simulink subsystem "station1"  (R2024b)
settings: Solver=VariableStepAuto  StartTime=0.0  StopTime=10.0  RelTol=1e-3
undefined symbols (not defined in the file): DiscIntNeverNeededParam, DPL1ph, h, Half, R3, ResistanceM, Rt4, simetran, Ts, Zm
libraries: ee_lib x102, fl_lib x54, nesl_utility x45, simulink x7
(part 3 of 3)

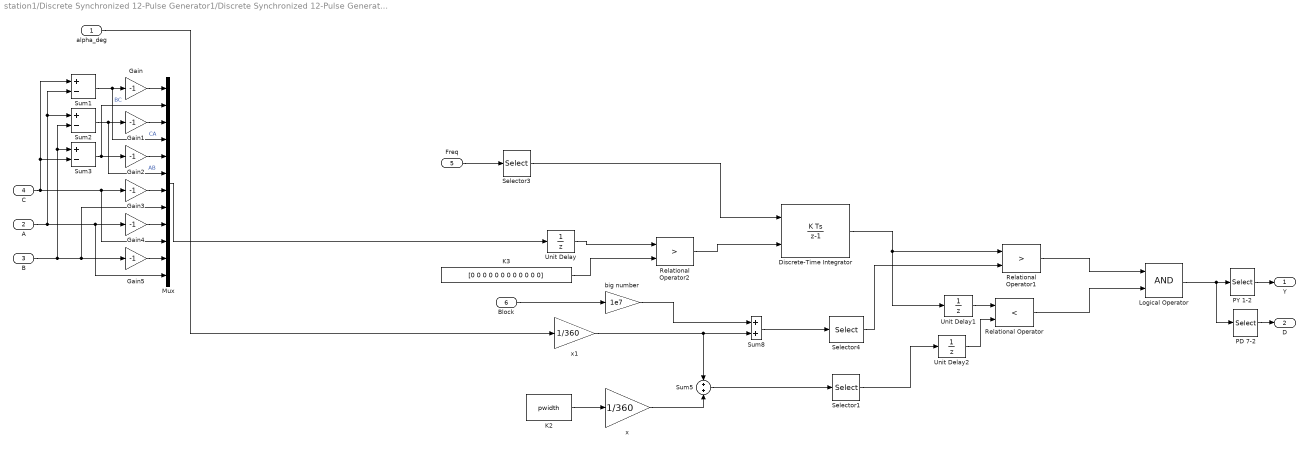
== system station1/Discrete Synchronized 12-Pulse Generator1/Discrete Synchronized 12-Pulse Generator2 ==
  alpha_deg : Inport
  A : Inport  Port=2
  B : Inport  Port=3
  C : Inport  Port=4
  Freq : Inport  Port=5
  Block : Inport  Port=6
  Discrete-Time Integrator : DiscreteIntegrator  ExternalReset=rising  SampleTime=Ts  ICPrevOutput=DiscIntNeverNeededParam  ICPrevScaledInput=DiscIntNeverNeededParam
  Gain{,1..5} (6 alike) : Gain  Gain=-1  SaturateOnIntegerOverflow=on  OutDataTypeStr=Inherit: Same as input  ParamDataTypeStr=Inherit: Same as input
  K2 : Constant  Value=pwidth
  K3 : Constant  Value=[0 0 0 0 0 0 0 0 0 0 0 0]
  Logical Operator : Logic  AllPortsSameDT=off  OutDataTypeStr=boolean
  Mux : Mux  Inputs=12
  PD 7-2 : Selector  InputPortWidth=12  IndexOptions=Index vector (dialog)  Indices=7:12  OutputSizes=1
  PY 1-2 : Selector  InputPortWidth=12  IndexOptions=Index vector (dialog)  Indices=1:6  OutputSizes=1
  Relational Operator : RelationalOperator  Operator=<  OutDataTypeStr=boolean  RndMeth=Simplest  InputSameDT=off
  Relational Operator1 : RelationalOperator  Operator=>  OutDataTypeStr=boolean  RndMeth=Simplest  InputSameDT=off
  Relational Operator2 : RelationalOperator  Operator=>  OutDataTypeStr=boolean  RndMeth=Simplest  InputSameDT=off
  Selector1 : Selector  InputPortWidth=1  IndexOptions=Index vector (dialog)  Indices=[1 1 1 1 1 1 1 1 1 1 1 1]  OutputSizes=1
  Selector3 : Selector  InputPortWidth=1  IndexOptions=Index vector (dialog)  Indices=[1 1 1 1 1 1 1 1 1 1 1 1]  OutputSizes=1
  Selector4 : Selector  InputPortWidth=1  IndexOptions=Index vector (dialog)  Indices=[1 1 1 1 1 1 1 1 1 1 1 1]  OutputSizes=1
  Sum1 : Sum  Inputs=+-  InputSameDT=on  SaturateOnIntegerOverflow=on  OutDataTypeStr=Inherit: Same as first input
  Sum2 : Sum  Inputs=+-  InputSameDT=on  SaturateOnIntegerOverflow=on  OutDataTypeStr=Inherit: Same as first input
  Sum3 : Sum  Inputs=+-  InputSameDT=on  SaturateOnIntegerOverflow=on  OutDataTypeStr=Inherit: Same as first input
  Sum5 : Sum  InputSameDT=on  SaturateOnIntegerOverflow=on  OutDataTypeStr=Inherit: Same as first input
  Sum8 : Sum  InputSameDT=on  SaturateOnIntegerOverflow=on  OutDataTypeStr=Inherit: Same as first input
  Unit Delay : UnitDelay  InitialCondition=-1  SampleTime=Ts  HasFrameUpgradeWarning=on
  Unit Delay1 : UnitDelay  InitialCondition=-1  SampleTime=Ts  HasFrameUpgradeWarning=on
  Unit Delay2 : UnitDelay  InitialCondition=-1  SampleTime=Ts  HasFrameUpgradeWarning=on
  big number : Gain  Gain=1e7  SaturateOnIntegerOverflow=on  OutDataTypeStr=Inherit: Same as input  ParamDataTypeStr=Inherit: Same as input
  x : Gain  Gain=1/360  SaturateOnIntegerOverflow=on  OutDataTypeStr=Inherit: Same as input  ParamDataTypeStr=Inherit: Same as input
  x1 : Gain  Gain=1/360  SaturateOnIntegerOverflow=on  OutDataTypeStr=Inherit: Same as input  ParamDataTypeStr=Inherit: Same as input
  Y : Outport  InitialOutput=0
  D : Outport  Port=2  InitialOutput=0
  wires:
  Unit Delay2/1 -> Relational Operator/2
  Unit Delay1/1 -> Relational Operator/1
  Freq/1 -> Selector3/1
  Gain2/1 -> Mux/5
  Gain1/1 -> Mux/3
  Gain/1 -> Mux/1
  Sum1/1 -> Gain/1, Mux/4  "CA"
  Sum2/1 -> Gain1/1, Mux/6  "AB"
  Sum3/1 -> Gain2/1, Mux/2  "BC"
  Gain3/1 -> Mux/7
  Gain4/1 -> Mux/9
  Gain5/1 -> Mux/11
  C/1 -> Gain3/1, Mux/10, Sum1/1, Sum3/2
  A/1 -> Gain4/1, Mux/12, Sum2/1, Sum1/2
  B/1 -> Gain5/1, Mux/8, Sum3/1, Sum2/2
  Block/1 -> big number/1
  Selector3/1 -> Discrete-Time Integrator/1
  big number/1 -> Sum8/1
  Selector1/1 -> Unit Delay2/1
  Logical Operator/1 -> PD 7-2/1, PY 1-2/1
  Sum5/1 -> Selector1/1
  Discrete-Time Integrator/1 -> Relational Operator1/1, Unit Delay1/1
  Mux/1 -> Unit Delay/1
  K3/1 -> Relational Operator2/2
  Relational Operator1/1 -> Logical Operator/1
  Relational Operator/1 -> Logical Operator/2
  x/1 -> Sum5/2
  K2/1 -> x/1
  Relational Operator2/1 -> Discrete-Time Integrator/2
  alpha_deg/1 -> x1/1
  Unit Delay/1 -> Relational Operator2/1
  Sum8/1 -> Selector4/1
  PD 7-2/1 -> D/1
  PY 1-2/1 -> Y/1
  x1/1 -> Sum8/2, Sum5/1
  Selector4/1 -> Relational Operator1/2

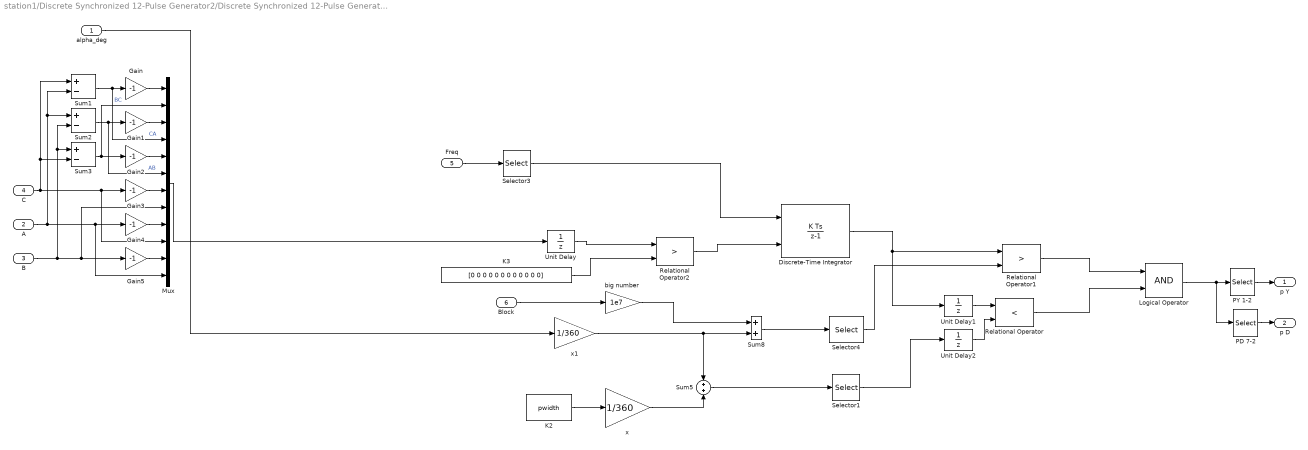
== system station1/Discrete Synchronized 12-Pulse Generator2/Discrete Synchronized 12-Pulse Generator2 ==
  alpha_deg : Inport
  A : Inport  Port=2
  B : Inport  Port=3
  C : Inport  Port=4
  Freq : Inport  Port=5
  Block : Inport  Port=6
  Discrete-Time Integrator : DiscreteIntegrator  ExternalReset=rising  SampleTime=Ts  ICPrevOutput=DiscIntNeverNeededParam  ICPrevScaledInput=DiscIntNeverNeededParam
  Gain{,1..5} (6 alike) : Gain  Gain=-1  SaturateOnIntegerOverflow=on  OutDataTypeStr=Inherit: Same as input  ParamDataTypeStr=Inherit: Same as input
  K2 : Constant  Value=pwidth
  K3 : Constant  Value=[0 0 0 0 0 0 0 0 0 0 0 0]
  Logical Operator : Logic  AllPortsSameDT=off  OutDataTypeStr=boolean
  Mux : Mux  Inputs=12
  PD 7-2 : Selector  InputPortWidth=12  IndexOptions=Index vector (dialog)  Indices=7:12  OutputSizes=1
  PY 1-2 : Selector  InputPortWidth=12  IndexOptions=Index vector (dialog)  Indices=1:6  OutputSizes=1
  Relational Operator : RelationalOperator  Operator=<  OutDataTypeStr=boolean  RndMeth=Simplest  InputSameDT=off
  Relational Operator1 : RelationalOperator  Operator=>  OutDataTypeStr=boolean  RndMeth=Simplest  InputSameDT=off
  Relational Operator2 : RelationalOperator  Operator=>  OutDataTypeStr=boolean  RndMeth=Simplest  InputSameDT=off
  Selector1 : Selector  InputPortWidth=1  IndexOptions=Index vector (dialog)  Indices=[1 1 1 1 1 1 1 1 1 1 1 1]  OutputSizes=1
  Selector3 : Selector  InputPortWidth=1  IndexOptions=Index vector (dialog)  Indices=[1 1 1 1 1 1 1 1 1 1 1 1]  OutputSizes=1
  Selector4 : Selector  InputPortWidth=1  IndexOptions=Index vector (dialog)  Indices=[1 1 1 1 1 1 1 1 1 1 1 1]  OutputSizes=1
  Sum1 : Sum  Inputs=+-  InputSameDT=on  SaturateOnIntegerOverflow=on  OutDataTypeStr=Inherit: Same as first input
  Sum2 : Sum  Inputs=+-  InputSameDT=on  SaturateOnIntegerOverflow=on  OutDataTypeStr=Inherit: Same as first input
  Sum3 : Sum  Inputs=+-  InputSameDT=on  SaturateOnIntegerOverflow=on  OutDataTypeStr=Inherit: Same as first input
  Sum5 : Sum  InputSameDT=on  SaturateOnIntegerOverflow=on  OutDataTypeStr=Inherit: Same as first input
  Sum8 : Sum  InputSameDT=on  SaturateOnIntegerOverflow=on  OutDataTypeStr=Inherit: Same as first input
  Unit Delay : UnitDelay  InitialCondition=-1  SampleTime=Ts  HasFrameUpgradeWarning=on
  Unit Delay1 : UnitDelay  InitialCondition=-1  SampleTime=Ts  HasFrameUpgradeWarning=on
  Unit Delay2 : UnitDelay  InitialCondition=-1  SampleTime=Ts  HasFrameUpgradeWarning=on
  big number : Gain  Gain=1e7  SaturateOnIntegerOverflow=on  OutDataTypeStr=Inherit: Same as input  ParamDataTypeStr=Inherit: Same as input
  x : Gain  Gain=1/360  SaturateOnIntegerOverflow=on  OutDataTypeStr=Inherit: Same as input  ParamDataTypeStr=Inherit: Same as input
  x1 : Gain  Gain=1/360  SaturateOnIntegerOverflow=on  OutDataTypeStr=Inherit: Same as input  ParamDataTypeStr=Inherit: Same as input
  p Y : Outport  InitialOutput=0
  p D : Outport  Port=2  InitialOutput=0
  wires:
  Selector4/1 -> Relational Operator1/2
  x1/1 -> Sum5/1, Sum8/2
  PY 1-2/1 -> p Y/1
  PD 7-2/1 -> p D/1
  Sum8/1 -> Selector4/1
  Unit Delay/1 -> Relational Operator2/1
  alpha_deg/1 -> x1/1
  Relational Operator2/1 -> Discrete-Time Integrator/2
  K2/1 -> x/1
  x/1 -> Sum5/2
  Relational Operator/1 -> Logical Operator/2
  Relational Operator1/1 -> Logical Operator/1
  K3/1 -> Relational Operator2/2
  Mux/1 -> Unit Delay/1
  Discrete-Time Integrator/1 -> Unit Delay1/1, Relational Operator1/1
  Sum5/1 -> Selector1/1
  Logical Operator/1 -> PY 1-2/1, PD 7-2/1
  Selector1/1 -> Unit Delay2/1
  big number/1 -> Sum8/1
  Selector3/1 -> Discrete-Time Integrator/1
  Block/1 -> big number/1
  B/1 -> Sum2/2, Sum3/1, Mux/8, Gain5/1
  A/1 -> Sum1/2, Sum2/1, Mux/12, Gain4/1
  C/1 -> Sum3/2, Sum1/1, Mux/10, Gain3/1
  Gain5/1 -> Mux/11
  Gain4/1 -> Mux/9
  Gain3/1 -> Mux/7
  Sum3/1 -> Mux/2, Gain2/1  "BC"
  Sum2/1 -> Mux/6, Gain1/1  "AB"
  Sum1/1 -> Mux/4, Gain/1  "CA"
  Gain/1 -> Mux/1
  Gain1/1 -> Mux/3
  Gain2/1 -> Mux/5
  Freq/1 -> Selector3/1
  Unit Delay1/1 -> Relational Operator/1
  Unit Delay2/1 -> Relational Operator/2

== system station1/Filters 60Hz8/High-pass filter ==
  CC : fl_lib/Electrical/Electrical Elements/Capacitor  c=C1 F  r=0 Ohm  g=0 1/Ohm  i_specify=off  i_priority=None  i=0 A  i_nominal_specify=off  i_nominal_value=1  i_nominal_unit=A  v_specify=off  v_priority=None  v=0 V  v_nominal_specify=off  v_nominal_value=1  v_nominal_unit=V  vc_specify=off  vc_priority=High  vc=0 V  vc_nominal_specify=off  vc_nominal_value=1  vc_nominal_unit=V
  CC1 : fl_lib/Electrical/Electrical Elements/Capacitor  c=C1 F  r=0 Ohm  g=0 1/Ohm  i_specify=off  i_priority=None  i=0 A  i_nominal_specify=off  i_nominal_value=1  i_nominal_unit=A  v_specify=off  v_priority=None  v=0 V  v_nominal_specify=off  v_nominal_value=1  v_nominal_unit=V  vc_specify=off  vc_priority=High  vc=0 V  vc_nominal_specify=off  vc_nominal_value=1  vc_nominal_unit=V
  CC2 : fl_lib/Electrical/Electrical Elements/Capacitor  c=C1 F  r=0 Ohm  g=0 1/Ohm  i_specify=off  i_priority=None  i=0 A  i_nominal_specify=off  i_nominal_value=1  i_nominal_unit=A  v_specify=off  v_priority=None  v=0 V  v_nominal_specify=off  v_nominal_value=1  v_nominal_unit=V  vc_specify=off  vc_priority=High  vc=0 V  vc_nominal_specify=off  vc_nominal_value=1  vc_nominal_unit=V
  Electrical Reference : fl_lib/Electrical/Electrical Elements/Electrical Reference
  Electrical Reference1 : fl_lib/Electrical/Electrical Elements/Electrical Reference
  Electrical Reference2 : fl_lib/Electrical/Electrical Elements/Electrical Reference
  Phase Splitter : ee_lib/Connectors & References/Phase Splitter
  RL parallel : fl_lib/Electrical/Electrical Elements/Inductor  l=L2 H  r=0 Ohm  g=1/R3 1/Ohm  i_specify=off  i_priority=None  i=0 A  i_nominal_specify=off  i_nominal_value=1  i_nominal_unit=A  v_specify=off  v_priority=None  v=0 V  v_nominal_specify=off  v_nominal_value=1  v_nominal_unit=V  i_L_specify=off  i_L_priority=High  i_L=0 A  i_L_nominal_specify=off  i_L_nominal_value=1  i_L_nominal_unit=A
  RL parallel1 : fl_lib/Electrical/Electrical Elements/Inductor  l=L2 H  r=0 Ohm  g=1/R3 1/Ohm  i_specify=off  i_priority=None  i=0 A  i_nominal_specify=off  i_nominal_value=1  i_nominal_unit=A  v_specify=off  v_priority=None  v=0 V  v_nominal_specify=off  v_nominal_value=1  v_nominal_unit=V  i_L_specify=off  i_L_priority=High  i_L=0 A  i_L_nominal_specify=off  i_L_nominal_value=1  i_L_nominal_unit=A
  RL parallel2 : fl_lib/Electrical/Electrical Elements/Inductor  l=L2 H  r=0 Ohm  g=1/R3 1/Ohm  i_specify=off  i_priority=None  i=0 A  i_nominal_specify=off  i_nominal_value=1  i_nominal_unit=A  v_specify=off  v_priority=None  v=0 V  v_nominal_specify=off  v_nominal_value=1  v_nominal_unit=V  i_L_specify=off  i_L_priority=High  i_L=0 A  i_L_nominal_specify=off  i_L_nominal_value=1  i_L_nominal_unit=A
  abc : PMIOPort  Side=Right
  connections:
  CC2/LConn1 -- Phase Splitter/RConn3
  CC/LConn1 -- Phase Splitter/RConn1
  Phase Splitter/RConn2 -- CC1/LConn1
  Phase Splitter/LConn1 -- abc/RConn1
  RL parallel/LConn1 -- CC/RConn1
  RL parallel/RConn1 -- Electrical Reference/LConn1
  CC1/RConn1 -- RL parallel1/LConn1
  RL parallel1/RConn1 -- Electrical Reference1/LConn1
  RL parallel2/RConn1 -- Electrical Reference2/LConn1
  CC2/RConn1 -- RL parallel2/LConn1

== system station1/Filters 60Hz8/tuned filter 11th ==
  Electrical Reference : fl_lib/Electrical/Electrical Elements/Electrical Reference
  Electrical Reference1 : fl_lib/Electrical/Electrical Elements/Electrical Reference
  Electrical Reference2 : fl_lib/Electrical/Electrical Elements/Electrical Reference
  Inductor : fl_lib/Electrical/Electrical Elements/Inductor  l=L1 H  r=R2 Ohm  g=1e-9 1/Ohm  i_specify=off  i_priority=None  i=0 A  i_nominal_specify=off  i_nominal_value=1  i_nominal_unit=A  v_specify=off  v_priority=None  v=0 V  v_nominal_specify=off  v_nominal_value=1  v_nominal_unit=V  i_L_specify=off  i_L_priority=High  i_L=0 A  i_L_nominal_specify=off  i_L_nominal_value=1  i_L_nominal_unit=A
  Inductor1 : fl_lib/Electrical/Electrical Elements/Inductor  l=L1 H  r=R2 Ohm  g=1e-9 1/Ohm  i_specify=off  i_priority=None  i=0 A  i_nominal_specify=off  i_nominal_value=1  i_nominal_unit=A  v_specify=off  v_priority=None  v=0 V  v_nominal_specify=off  v_nominal_value=1  v_nominal_unit=V  i_L_specify=off  i_L_priority=High  i_L=0 A  i_L_nominal_specify=off  i_L_nominal_value=1  i_L_nominal_unit=A
  Inductor2 : fl_lib/Electrical/Electrical Elements/Inductor  l=L1 H  r=R2 Ohm  g=1e-9 1/Ohm  i_specify=off  i_priority=None  i=0 A  i_nominal_specify=off  i_nominal_value=1  i_nominal_unit=A  v_specify=off  v_priority=None  v=0 V  v_nominal_specify=off  v_nominal_value=1  v_nominal_unit=V  i_L_specify=off  i_L_priority=High  i_L=0 A  i_L_nominal_specify=off  i_L_nominal_value=1  i_L_nominal_unit=A
  Phase Splitter : ee_lib/Connectors & References/Phase Splitter
  RC : fl_lib/Electrical/Electrical Elements/Capacitor  c=C1 F  r=0 Ohm  g=0 1/Ohm  i_specify=off  i_priority=None  i=0 A  i_nominal_specify=off  i_nominal_value=1  i_nominal_unit=A  v_specify=off  v_priority=None  v=0 V  v_nominal_specify=off  v_nominal_value=1  v_nominal_unit=V  vc_specify=off  vc_priority=High  vc=0 V  vc_nominal_specify=off  vc_nominal_value=1  vc_nominal_unit=V
  RC1 : fl_lib/Electrical/Electrical Elements/Capacitor  c=C1 F  r=0 Ohm  g=0 1/Ohm  i_specify=off  i_priority=None  i=0 A  i_nominal_specify=off  i_nominal_value=1  i_nominal_unit=A  v_specify=off  v_priority=None  v=0 V  v_nominal_specify=off  v_nominal_value=1  v_nominal_unit=V  vc_specify=off  vc_priority=High  vc=0 V  vc_nominal_specify=off  vc_nominal_value=1  vc_nominal_unit=V
  RC2 : fl_lib/Electrical/Electrical Elements/Capacitor  c=C1 F  r=0 Ohm  g=0 1/Ohm  i_specify=off  i_priority=None  i=0 A  i_nominal_specify=off  i_nominal_value=1  i_nominal_unit=A  v_specify=off  v_priority=None  v=0 V  v_nominal_specify=off  v_nominal_value=1  v_nominal_unit=V  vc_specify=off  vc_priority=High  vc=0 V  vc_nominal_specify=off  vc_nominal_value=1  vc_nominal_unit=V
  abc : PMIOPort  Side=Right
  connections:
  Phase Splitter/LConn1 -- abc/RConn1
  RC2/LConn1 -- Phase Splitter/RConn3
  RC/LConn1 -- Phase Splitter/RConn1
  Phase Splitter/RConn2 -- RC1/LConn1
  RC2/RConn1 -- Inductor2/LConn1
  Inductor2/RConn1 -- Electrical Reference2/LConn1
  Inductor1/RConn1 -- Electrical Reference1/LConn1
  RC1/RConn1 -- Inductor1/LConn1
  Inductor/RConn1 -- Electrical Reference/LConn1
  Inductor/LConn1 -- RC/RConn1

== system station1/Filters 60Hz8/tuned filter 13th ==
  Electrical Reference : fl_lib/Electrical/Electrical Elements/Electrical Reference
  Electrical Reference1 : fl_lib/Electrical/Electrical Elements/Electrical Reference
  Electrical Reference2 : fl_lib/Electrical/Electrical Elements/Electrical Reference
  Inductor : fl_lib/Electrical/Electrical Elements/Inductor  l=L1 H  r=R2 Ohm  g=1e-9 1/Ohm  i_specify=off  i_priority=None  i=0 A  i_nominal_specify=off  i_nominal_value=1  i_nominal_unit=A  v_specify=off  v_priority=None  v=0 V  v_nominal_specify=off  v_nominal_value=1  v_nominal_unit=V  i_L_specify=off  i_L_priority=High  i_L=0 A  i_L_nominal_specify=off  i_L_nominal_value=1  i_L_nominal_unit=A
  Inductor1 : fl_lib/Electrical/Electrical Elements/Inductor  l=L1 H  r=R2 Ohm  g=1e-9 1/Ohm  i_specify=off  i_priority=None  i=0 A  i_nominal_specify=off  i_nominal_value=1  i_nominal_unit=A  v_specify=off  v_priority=None  v=0 V  v_nominal_specify=off  v_nominal_value=1  v_nominal_unit=V  i_L_specify=off  i_L_priority=High  i_L=0 A  i_L_nominal_specify=off  i_L_nominal_value=1  i_L_nominal_unit=A
  Inductor2 : fl_lib/Electrical/Electrical Elements/Inductor  l=L1 H  r=R2 Ohm  g=1e-9 1/Ohm  i_specify=off  i_priority=None  i=0 A  i_nominal_specify=off  i_nominal_value=1  i_nominal_unit=A  v_specify=off  v_priority=None  v=0 V  v_nominal_specify=off  v_nominal_value=1  v_nominal_unit=V  i_L_specify=off  i_L_priority=High  i_L=0 A  i_L_nominal_specify=off  i_L_nominal_value=1  i_L_nominal_unit=A
  Phase Splitter : ee_lib/Connectors & References/Phase Splitter
  RC : fl_lib/Electrical/Electrical Elements/Capacitor  c=C1 F  r=0 Ohm  g=0 1/Ohm  i_specify=off  i_priority=None  i=0 A  i_nominal_specify=off  i_nominal_value=1  i_nominal_unit=A  v_specify=off  v_priority=None  v=0 V  v_nominal_specify=off  v_nominal_value=1  v_nominal_unit=V  vc_specify=off  vc_priority=High  vc=0 V  vc_nominal_specify=off  vc_nominal_value=1  vc_nominal_unit=V
  RC1 : fl_lib/Electrical/Electrical Elements/Capacitor  c=C1 F  r=0 Ohm  g=0 1/Ohm  i_specify=off  i_priority=None  i=0 A  i_nominal_specify=off  i_nominal_value=1  i_nominal_unit=A  v_specify=off  v_priority=None  v=0 V  v_nominal_specify=off  v_nominal_value=1  v_nominal_unit=V  vc_specify=off  vc_priority=High  vc=0 V  vc_nominal_specify=off  vc_nominal_value=1  vc_nominal_unit=V
  RC2 : fl_lib/Electrical/Electrical Elements/Capacitor  c=C1 F  r=0 Ohm  g=0 1/Ohm  i_specify=off  i_priority=None  i=0 A  i_nominal_specify=off  i_nominal_value=1  i_nominal_unit=A  v_specify=off  v_priority=None  v=0 V  v_nominal_specify=off  v_nominal_value=1  v_nominal_unit=V  vc_specify=off  vc_priority=High  vc=0 V  vc_nominal_specify=off  vc_nominal_value=1  vc_nominal_unit=V
  abc : PMIOPort  Side=Right
  connections:
  Inductor/LConn1 -- RC/RConn1
  Inductor/RConn1 -- Electrical Reference/LConn1
  RC1/RConn1 -- Inductor1/LConn1
  Inductor1/RConn1 -- Electrical Reference1/LConn1
  Inductor2/RConn1 -- Electrical Reference2/LConn1
  RC2/RConn1 -- Inductor2/LConn1
  Phase Splitter/RConn2 -- RC1/LConn1
  RC/LConn1 -- Phase Splitter/RConn1
  RC2/LConn1 -- Phase Splitter/RConn3
  Phase Splitter/LConn1 -- abc/RConn1

== system station1/Half-DPL1ph/Simscape ==
  Electrical Reference1 : fl_lib/Electrical/Electrical Elements/Electrical Reference
  PS-S : nesl_utility/PS-Simulink Converter  PhysicalDomain=network_engine_domain  SubClassName=ps_output  LeftPortType=input  RightPortType=output  PseudoPeriodic=off  Frequencies=[]  VectorFormat=1-D array  Unit=V  AffineConversion=off
  Voltage Sensor : fl_lib/Electrical/Electrical Sensors/Voltage Sensor
  V : PMIOPort  Side=Left
  Out : Outport  VectorParamsAs1DForOutWhenUnconnected=off
  wires:
  PS-S/1 -> Out/1  "voltage"
  connections:
  PS-S/LConn1 -- Voltage Sensor/RConn1
  V/RConn1 -- Voltage Sensor/LConn1
  Electrical Reference1/LConn1 -- Voltage Sensor/RConn2

== system station1/Half-DPL1ph/Voltage Source ==
  I : Inport
  Controlled Current Source1 : fl_lib/Electrical/Electrical Sources/Controlled Current Source
  Simulink-PS Converter : nesl_utility/Simulink-PS Converter  PhysicalDomain=network_engine_domain  SubClassName=ps_input  LeftPortType=input  RightPortType=output  PseudoPeriodic=off  Frequencies=[]  NoiseDistribution=none  NoiseParameters=[]  Unit=1  AffineConversion=off  FilteringAndDerivatives=zero  SimscapeFilterOrder=1  InputFilterTimeConstant=.001  UdotUserProvided=0
  + : PMIOPort  Side=Right
  - : PMIOPort  Port=2  Side=Right
  wires:
  I/1 -> Simulink-PS Converter/1
  connections:
  Controlled Current Source1/RConn1 -- Simulink-PS Converter/RConn1
  Controlled Current Source1/RConn2 -- -/RConn1
  Controlled Current Source1/LConn1 -- +/RConn1

== system station1/Half-DPL1ph/dplmodel ==
  v : Inport
  hist_in : Inport  Port=2
  (1+h)/Z : Gain  Gain=(1+h)./(Zm+Rt4)  SaturateOnIntegerOverflow=on  OutDataTypeStr=Inherit: Same as input  ParamDataTypeStr=Inherit: Same as input
  Gain4 : Gain  Gain=(1+h)/2  SaturateOnIntegerOverflow=on  OutDataTypeStr=Inherit: Same as input  ParamDataTypeStr=Inherit: Same as input
  Gain6 : Gain  Gain=(1-h)/2  SaturateOnIntegerOverflow=on  OutDataTypeStr=Inherit: Same as input  ParamDataTypeStr=Inherit: Same as input
  Gain9 : Gain  Gain=h  SaturateOnIntegerOverflow=on  OutDataTypeStr=Inherit: Same as input  ParamDataTypeStr=Inherit: Same as input
  Sum1 : Sum  Inputs=-+  InputSameDT=on  SaturateOnIntegerOverflow=on  OutDataTypeStr=Inherit: Same as first input
  Sum3 : Sum  InputSameDT=on  SaturateOnIntegerOverflow=on  OutDataTypeStr=Inherit: Same as first input
  derlay : Subsystem
  i : Outport  InitialOutput=0  VectorParamsAs1DForOutWhenUnconnected=off
  hist_out : Outport  Port=2  VectorParamsAs1DForOutWhenUnconnected=off
  wires:
  Sum3/1 -> i/1, Gain9/1
  v/1 -> (1+h)/Z/1
  Gain4/1 -> hist_out/1
  Gain9/1 -> Sum1/1
  (1+h)/Z/1 -> Sum1/2
  Gain6/1 -> Sum3/1
  hist_in/1 -> Sum3/2
  derlay/1(Out1) -> Gain4/1, Gain6/1
  Sum1/1 -> derlay/1(In1)

== system station1/Half-DPL1ph1/Simscape ==
  Electrical Reference1 : fl_lib/Electrical/Electrical Elements/Electrical Reference
  PS-S : nesl_utility/PS-Simulink Converter  PhysicalDomain=network_engine_domain  SubClassName=ps_output  LeftPortType=input  RightPortType=output  PseudoPeriodic=off  Frequencies=[]  VectorFormat=1-D array  Unit=V  AffineConversion=off
  Voltage Sensor : fl_lib/Electrical/Electrical Sensors/Voltage Sensor
  V : PMIOPort  Side=Left
  Out : Outport  VectorParamsAs1DForOutWhenUnconnected=off
  wires:
  PS-S/1 -> Out/1  "voltage"
  connections:
  Electrical Reference1/LConn1 -- Voltage Sensor/RConn2
  V/RConn1 -- Voltage Sensor/LConn1
  PS-S/LConn1 -- Voltage Sensor/RConn1

== system station1/Half-DPL1ph1/Voltage Source ==
  I : Inport
  Controlled Current Source1 : fl_lib/Electrical/Electrical Sources/Controlled Current Source
  Simulink-PS Converter : nesl_utility/Simulink-PS Converter  PhysicalDomain=network_engine_domain  SubClassName=ps_input  LeftPortType=input  RightPortType=output  PseudoPeriodic=off  Frequencies=[]  NoiseDistribution=none  NoiseParameters=[]  Unit=1  AffineConversion=off  FilteringAndDerivatives=zero  SimscapeFilterOrder=1  InputFilterTimeConstant=.001  UdotUserProvided=0
  + : PMIOPort  Side=Right
  - : PMIOPort  Port=2  Side=Right
  wires:
  I/1 -> Simulink-PS Converter/1
  connections:
  Controlled Current Source1/LConn1 -- +/RConn1
  Controlled Current Source1/RConn2 -- -/RConn1
  Controlled Current Source1/RConn1 -- Simulink-PS Converter/RConn1

== system station1/Half-DPL1ph1/dplmodel ==
  v : Inport
  hist_in : Inport  Port=2
  (1+h)/Z : Gain  Gain=(1+h)./(Zm+Rt4)  SaturateOnIntegerOverflow=on  OutDataTypeStr=Inherit: Same as input  ParamDataTypeStr=Inherit: Same as input
  Gain4 : Gain  Gain=(1+h)/2  SaturateOnIntegerOverflow=on  OutDataTypeStr=Inherit: Same as input  ParamDataTypeStr=Inherit: Same as input
  Gain6 : Gain  Gain=(1-h)/2  SaturateOnIntegerOverflow=on  OutDataTypeStr=Inherit: Same as input  ParamDataTypeStr=Inherit: Same as input
  Gain9 : Gain  Gain=h  SaturateOnIntegerOverflow=on  OutDataTypeStr=Inherit: Same as input  ParamDataTypeStr=Inherit: Same as input
  Sum1 : Sum  Inputs=-+  InputSameDT=on  SaturateOnIntegerOverflow=on  OutDataTypeStr=Inherit: Same as first input
  Sum3 : Sum  InputSameDT=on  SaturateOnIntegerOverflow=on  OutDataTypeStr=Inherit: Same as first input
  derlay : Subsystem
  i : Outport  InitialOutput=0  VectorParamsAs1DForOutWhenUnconnected=off
  hist_out : Outport  Port=2  VectorParamsAs1DForOutWhenUnconnected=off
  wires:
  Sum1/1 -> derlay/1(In1)
  derlay/1(Out1) -> Gain6/1, Gain4/1
  hist_in/1 -> Sum3/2
  Gain6/1 -> Sum3/1
  (1+h)/Z/1 -> Sum1/2
  Gain9/1 -> Sum1/1
  Gain4/1 -> hist_out/1
  v/1 -> (1+h)/Z/1
  Sum3/1 -> Gain9/1, i/1

== system station1/Half-DPL1ph/dplmodel/derlay ==
  In1 : Inport
  Add : Sum
  Delay1 : Delay  DelayLength=delay(1)
  Gain : Gain  Gain=remd
  Gain1 : Gain  Gain=1-remd
  Unit Delay1 : UnitDelay  SampleTime=Ts  HasFrameUpgradeWarning=on
  Out1 : Outport
  wires:
  In1/1 -> Delay1/1
  Gain/1 -> Add/1
  Gain1/1 -> Add/2
  Unit Delay1/1 -> Gain/1
  Add/1 -> Out1/1
  Delay1/1 -> Gain1/1, Unit Delay1/1

== system station1/Half-DPL1ph1/dplmodel/derlay ==
  In1 : Inport
  Add : Sum
  Delay1 : Delay  DelayLength=delay(1)
  Gain : Gain  Gain=remd
  Gain1 : Gain  Gain=1-remd
  Unit Delay1 : UnitDelay  SampleTime=Ts  HasFrameUpgradeWarning=on
  Out1 : Outport
  wires:
  Delay1/1 -> Unit Delay1/1, Gain1/1
  Add/1 -> Out1/1
  Unit Delay1/1 -> Gain/1
  Gain1/1 -> Add/2
  Gain/1 -> Add/1
  In1/1 -> Delay1/1
